simulink model "IDlorenz"  (R2020b)
settings: Solver=FixedStepAuto  StartTime=0.0  StopTime=7.9  FixedStep=0.001  RelTol=1e-3
libraries: simulink x1
settings Model: Creator=chen  LastModifiedBy=chen
settings DataIOCC: ExternalInput=poscmd,velcmd,friction  LoadExternalInput=on

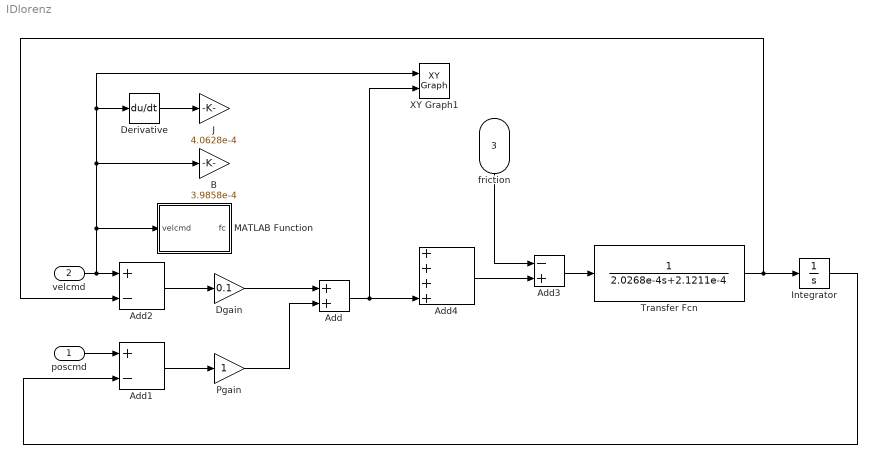
== system IDlorenz ==
  poscmd : Inport
  velcmd : Inport  Port=2
  friction : Inport  Port=3  PortDimensions=[1]  SampleTime=0.001
  Add : Sum
  Add1 : Sum  Inputs=+-
  Add2 : Sum  Inputs=+-
  Add3 : Sum  Inputs=-+
  Add4 : Sum  Inputs=++++
  B : Gain  Gain=3.9858e-4
  Derivative : Derivative
  Dgain : Gain  Gain=0.1
  Integrator : Integrator
  J : Gain  Gain=4.0628e-4
  MATLAB Function : MATLAB Function  TreatAsAtomicUnit=on
  Pgain : Gain
  Transfer Fcn : TransferFcn  Denominator=[2.0268e-4 ,2.1211e-4]
  XY Graph1 : simulink/Sinks/XY Graph  xmin=-60  xmax=60  ymin=-0.07  ymax=0.07  st=-1
  wires:
  Transfer Fcn/1 -> Add2/2, Integrator/1
  friction/1 -> Add3/1
  Add3/1 -> Transfer Fcn/1
  Add4/1 -> Add3/2
  Derivative/1 -> J/1
  poscmd/1 -> Add1/1
  Integrator/1 -> Add1/2
  velcmd/1 -> XY Graph1/1, Derivative/1, B/1, MATLAB Function/1(velcmd), Add2/1
  Add2/1 -> Dgain/1
  Dgain/1 -> Add/1
  Add1/1 -> Pgain/1
  Pgain/1 -> Add/2
  Add/1 -> XY Graph1/2, Add4/4

== matlab function IDlorenz/MATLAB Function ==
  data: velcmd input; fc output
function fc = fcn(velcmd)
    if velcmd >= 1.0
        fc = 0.0237;
    elseif velcmd < -1.38
        fc = -0.0307;
    else
        fc = 0;
    end
end
